simulink model "ad_fplib"  (R2015b)
settings: Solver=FixedStepDiscrete  SolverMode=SingleTasking  StartTime=0.0  StopTime=1  RelTol=1e-3
settings Model: Creator=amatsumo  LastModifiedBy=amatsumo
settings DataIOCC: SaveFormat=Array  SignalLoggingSaveFormat=ModelDataLogs  SaveOutput=off  SignalLogging=off  SaveTime=off
settings OptimizationCC: BlockReduction=off  ConditionallyExecuteInputs=off  DefaultParameterBehavior=Inlined  ExpressionDepthLimit=2147483647
settings DebuggingCC: AlgebraicLoopMsg=error  UnderspecifiedInitializationDetection=Classic  MergeDetectMultiDrivingBlocksExec=none  SolverPrmCheckMsg=warning  InheritedTsInSrcMsg=none  SingleTaskRateTransMsg=error  FcnCallInpInsideContextMsg=EnableAllAsWarning  StateNameClashWarn=warning
settings HardwareCC: ProdBitPerPointer=32  ProdLargestAtomicFloat=None  ProdIntDivRoundTo=Undefined  ProdEndianess=Unspecified  ProdWordSize=32  ProdHWDeviceType=ASIC/FPGA->ASIC/FPGA  ProdEqTarget=off
settings GRTTargetCC: GeneratePreprocessorConditionals=Disable all
settings ConfigComp: CovModelRefEnable=Off  CovSFcnEnable=off

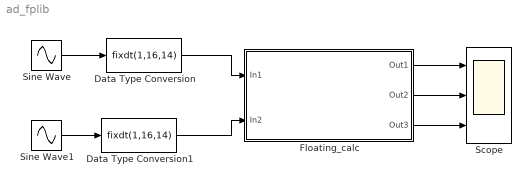
== system ad_fplib ==
  Data Type Conversion : DataTypeConversion  OutDataTypeStr=fixdt(1,16,14)
  Data Type Conversion1 : DataTypeConversion  OutDataTypeStr=fixdt(1,16,14)
  Floating_calc : Subsystem
  Scope : Scope  NumInputPorts=3
  Sine Wave : Sin  Frequency=2*pi*7  SampleTime=1/1000
  Sine Wave1 : Sin  Frequency=2*pi*10  SampleTime=1/1000
  wires:
  Sine Wave/1 -> Data Type Conversion/1
  Sine Wave1/1 -> Data Type Conversion1/1
  Data Type Conversion/1 -> Floating_calc/1(In1)
  Data Type Conversion1/1 -> Floating_calc/2(In2)
  Floating_calc/1(Out1) -> Scope/1
  Floating_calc/2(Out2) -> Scope/2
  Floating_calc/3(Out3) -> Scope/3

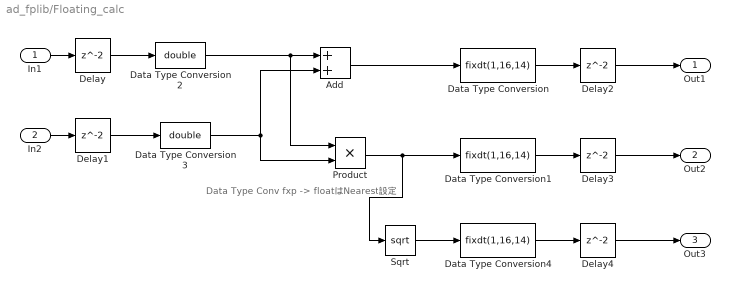
== system ad_fplib/Floating_calc ==
  note: Data Type Conv fxp -> float はNearest設定
  In1 : Inport
  In2 : Inport  Port=2
  Add : Sum
  Data Type Conversion : DataTypeConversion  OutDataTypeStr=fixdt(1,16,14)  RndMeth=Nearest
  Data Type Conversion1 : DataTypeConversion  OutDataTypeStr=fixdt(1,16,14)  RndMeth=Nearest
  Data Type Conversion2 : DataTypeConversion  OutDataTypeStr=double  RndMeth=Nearest
  Data Type Conversion3 : DataTypeConversion  OutDataTypeStr=double  RndMeth=Nearest
  Data Type Conversion4 : DataTypeConversion  OutDataTypeStr=fixdt(1,16,14)  RndMeth=Nearest
  Delay{,1..4} (5 alike) : Delay
  Product : Product  RndMeth=Zero
  Sqrt : Sqrt  OutputSignalType=real  SaturateOnIntegerOverflow=on
  Out1 : Outport
  Out2 : Outport  Port=2
  Out3 : Outport  Port=3
  wires:
  Delay/1 -> Data Type Conversion2/1
  Delay1/1 -> Data Type Conversion3/1
  Data Type Conversion2/1 -> Add/1, Product/1
  Data Type Conversion3/1 -> Add/2, Product/2
  Add/1 -> Data Type Conversion/1
  In1/1 -> Delay/1
  Delay2/1 -> Out1/1
  In2/1 -> Delay1/1
  Delay3/1 -> Out2/1
  Data Type Conversion/1 -> Delay2/1
  Data Type Conversion1/1 -> Delay3/1
  Data Type Conversion4/1 -> Delay4/1
  Delay4/1 -> Out3/1
  Sqrt/1 -> Data Type Conversion4/1
  Product/1 -> Sqrt/1, Data Type Conversion1/1
